simulink model "impedanceControl2012b"  (Simulink 8.0)
settings: Solver=FixedStepDiscrete  StartTime=0.0  StopTime=CONFIG.SIMULATION_TIME  FixedStep=Ts  RelTol=1e-3
InitFcn:
  | cd(fileparts(which(bdroot)));
  | init_impedanceControl;
values from neighbouring files (symbols this model uses):
  GRAV_COMP = 1    [init_impedanceControl.m]
  MOVING = 0    [init_impedanceControl.m]
undefined symbols (not defined in the file or in its folder): AMPLS, FREQS, Kd, Kp, ROBOT_DOF
libraries: WBToolboxLibrary x10
settings Model: Creator=daniele  LastModifiedBy=gnava
settings DataIOCC: SignalLoggingSaveFormat=ModelDataLogs
settings OptimizationCC: ExpressionDepthLimit=128
settings DebuggingCC: UnderspecifiedInitializationDetection=Simplified  MergeDetectMultiDrivingBlocksExec=error  MultiTaskDSMMsg=warning  MultiTaskCondExecSysMsg=none  FrameProcessingCompatibilityMsg=error  StateNameClashWarn=none  StrictBusMsg=ErrorOnBusTreatedAsVector
settings CodeAppCC: CustomSymbolStrType=$N$R$M_T
settings GRTTargetCC: CodeReplacementLibrary=C89/C90 (ANSI)

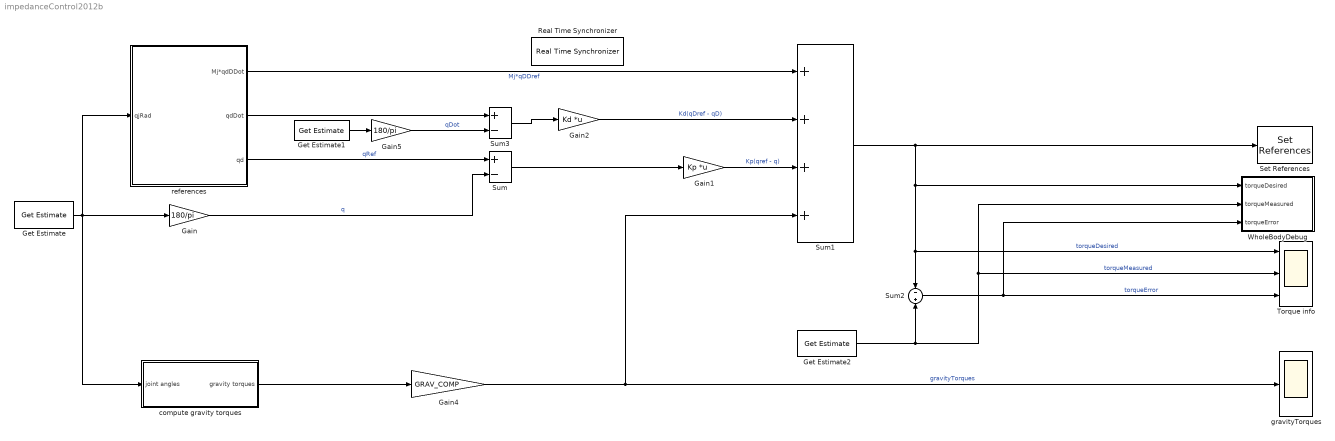
== system impedanceControl2012b ==
  Gain : Gain  Gain=180/pi
  Gain1 : Gain  Gain=Kp  Multiplication=Matrix(K*u)
  Gain2 : Gain  Gain=Kd  Multiplication=Matrix(K*u)
  Gain4 : Gain  Gain=GRAV_COMP
  Gain5 : Gain  Gain=180/pi
  Get Estimate : WBToolboxLibrary/wholeBodyStates/Get Estimate  estimateType=Joints Position  robotName=WBT_robotName  localName=WBT_modelName  wbiFile=WBT_wbiFilename  wbiList=WBT_wbiList
  Get Estimate1 : WBToolboxLibrary/wholeBodyStates/Get Estimate  estimateType=Joints Velocity  robotName=WBT_robotName  localName=WBT_modelName  wbiFile=WBT_wbiFilename  wbiList=WBT_wbiList
  Get Estimate2 : WBToolboxLibrary/wholeBodyStates/Get Estimate  estimateType=Joints Torque  robotName=WBT_robotName  localName=WBT_modelName  wbiFile=WBT_wbiFilename  wbiList=WBT_wbiList
  Real Time Synchronizer : WBToolboxLibrary/Utilities/Real Time Synchronizer  period=0.01
  Set References : WBToolboxLibrary/wholeBodyActuators/Set References  controlType=Torque  robotName=WBT_robotName  localName=WBT_modelName  wbiFile=WBT_wbiFilename  wbiList=WBT_wbiList
  Sum : Sum  Inputs=+-
  Sum1 : Sum  Inputs=++++
  Sum2 : Sum  Inputs=-|+
  Sum3 : Sum  Inputs=+-
  Torque info : Scope  NumInputPorts=3
      settings: TimeRange=20  ShowLegends=on  MaxDataPoints=5000  SaveToWorkspace=off  SaveName=ScopeData  YMin=-20.93013~-24.21652~-4.0063  YMax=5.78387~6.06845~4.66596  SampleTime=-1  DataFormat=Array
  WholeBodyDebug : Subsystem
  compute gravity torques : Subsystem
  gravityTorques : Scope
      settings: TimeRange=20  ShowLegends=on  MaxDataPoints=5000  SaveToWorkspace=off  YMin=-21.44461  YMax=11.35993  SampleTime=-1  DataFormat=Array
  references : Subsystem
  wires:
  Gain/1 -> Sum/2  "q"
  Sum/1 -> Gain1/1
  Gain1/1 -> Sum1/3  "Kp(qref - q)"
  Gain2/1 -> Sum1/2  "Kd(qDref - qD)"
  Get Estimate/1 -> compute gravity torques/1(joint angles), Gain/1, references/1(qjRad)
  Get Estimate2/1 -> WholeBodyDebug/2(torqueMeasured), Torque info/2, Sum2/2  "torqueMeasured"
  Sum2/1 -> WholeBodyDebug/3(torqueError), Torque info/3  "torqueError"
  references/3(" qd") -> Sum/1  "qRef"
  Gain5/1 -> Sum3/2  "qDot"
  Sum3/1 -> Gain2/1
  references/2(qdDot) -> Sum3/1
  references/1(Mj*qdDDot) -> Sum1/1  "Mj*qDDref"
  Gain4/1 -> Sum1/4, gravityTorques/1  "gravityTorques"
  Get Estimate1/1 -> Gain5/1
  compute gravity torques/1(gravity torques) -> Gain4/1
  Sum1/1 -> WholeBodyDebug/1(torqueDesired), Sum2/1, Torque info/1, Set References/1  "torqueDesired"

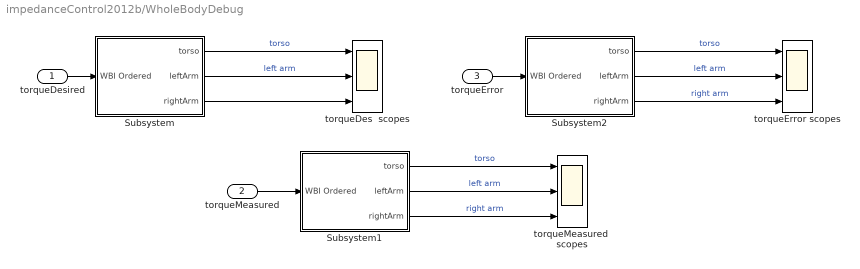
== system impedanceControl2012b/WholeBodyDebug ==
  torqueDesired : Inport
  torqueMeasured : Inport  Port=2
  torqueError : Inport  Port=3
  Subsystem : Subsystem
  Subsystem1 : Subsystem
  Subsystem2 : Subsystem
  torqueDes  scopes : Scope  NumInputPorts=3
      settings: TimeRange=60  ShowLegends=on  MaxDataPoints=5000  SaveToWorkspace=off  YMin=-21.03095~-3.42501~-3.44387  YMax=3.37527~2.67817~2.71878  SampleTime=-1
  "torqueError scopes  " : Scope  NumInputPorts=3
      settings: TimeRange=60  ShowLegends=on  MaxDataPoints=5000  SaveToWorkspace=off  SaveName=ScopeData3  YMin=-1.90536~-1.57907~-1.83653  YMax=7.25518~2.44036~2.59185  SampleTime=-1
  "torqueMeasured  scopes  " : Scope  NumInputPorts=3
      settings: TimeRange=60  ShowLegends=on  MaxDataPoints=5000  SaveToWorkspace=off  SaveName=ScopeData2  YMin=-12.98042~-3.01711~-2.9728  YMax=-3.60419~2.37899~2.11612  SampleTime=-1
  wires:
  torqueMeasured/1 -> Subsystem1/1(WBI Ordered)
  torqueError/1 -> Subsystem2/1(WBI Ordered)
  torqueDesired/1 -> Subsystem/1(WBI Ordered)
  Subsystem/1(torso) -> torqueDes  scopes/1  "torso"
  Subsystem/2(leftArm) -> torqueDes  scopes/2  "left arm"
  Subsystem1/1(torso) -> "torqueMeasured  scopes  "/1  "torso"
  Subsystem1/2(leftArm) -> "torqueMeasured  scopes  "/2  "left arm"
  Subsystem1/3(rightArm) -> "torqueMeasured  scopes  "/3  "right arm"
  Subsystem2/1(torso) -> "torqueError scopes  "/1  "torso"
  Subsystem2/2(leftArm) -> "torqueError scopes  "/2  "left arm"
  Subsystem2/3(rightArm) -> "torqueError scopes  "/3  "right arm"
  Subsystem/3(rightArm) -> torqueDes  scopes/3

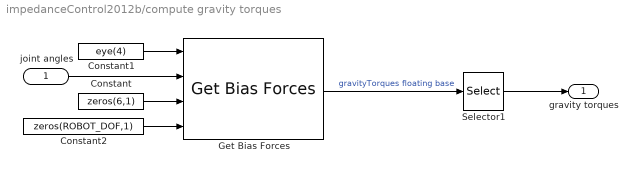
== system impedanceControl2012b/compute gravity torques ==
  joint angles : Inport
  Constant : Constant  Value=zeros(6,1)
  Constant1 : Constant  Value=eye(4)
  Constant2 : Constant  Value=zeros(ROBOT_DOF,1)
  Get Bias Forces : WBToolboxLibrary/wholeBodyModel/Dynamics/Get Bias Forces  robotName=WBT_robotName  localName=WBT_modelName  wbiFile=WBT_wbiFilename  wbiList=WBT_wbiList  explicitGravity=off
  Selector1 : Selector  InputPortWidth=ROBOT_DOF+6  IndexOptions=Index vector (dialog)  Indices=[7:ROBOT_DOF+6]  OutputSizes=1
  gravity torques : Outport
  wires:
  Selector1/1 -> gravity torques/1
  Constant1/1 -> Get Bias Forces/1
  Constant2/1 -> Get Bias Forces/4
  joint angles/1 -> Get Bias Forces/2
  Constant/1 -> Get Bias Forces/3
  Get Bias Forces/1 -> Selector1/1  "gravityTorques floating base"

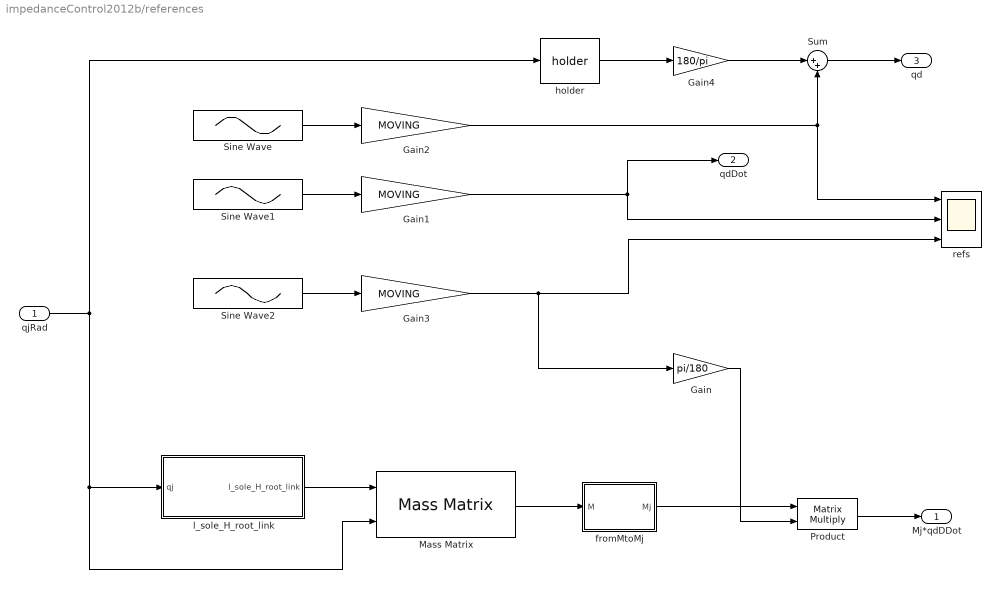
== system impedanceControl2012b/references ==
  qjRad : Inport
  Gain : Gain  Gain=pi/180
  Gain1 : Gain  Gain=MOVING
  Gain2 : Gain  Gain=MOVING
  Gain3 : Gain  Gain=MOVING
  Gain4 : Gain  Gain=180/pi
  Mass Matrix : WBToolboxLibrary/wholeBodyModel/Dynamics/Mass Matrix  robotName=WBT_robotName  localName=WBT_modelName  wbiFile=WBT_wbiFilename  wbiList=WBT_wbiList
  Product : Product  Multiplication=Matrix(*)
  Sine Wave : Sin  Amplitude=AMPLS  Frequency=FREQS*2*pi  SampleTime=0
  Sine Wave1 : Sin  Amplitude=AMPLS.*FREQS*2*pi  Frequency=FREQS*2*pi  Phase=pi/2  SampleTime=0
  Sine Wave2 : Sin  Amplitude=-AMPLS.*(FREQS*2*pi).^2  Frequency=FREQS*2*pi  SampleTime=0
  Sum : Sum  Inputs=|++
  fromMtoMj : MATLAB Function  TreatAsAtomicUnit=on
      settings: PermitHierarchicalResolution=ParametersOnly
  "holder " : WBToolboxLibrary/Utilities/holder 
  l_sole_H_root_link : Subsystem
  refs : Scope  NumInputPorts=3
      settings: TimeRange=70  ShowLegends=on  MaxDataPoints=5000  SaveToWorkspace=off  SaveName=ScopeData2  YMin=-5~-5~-5  YMax=4~5~5  SampleTime=-1  DataFormat=Array
  Mj*qdDDot : Outport
  qdDot : Outport  Port=2
  " qd" : Outport  Port=3
  wires:
  Sine Wave/1 -> Gain2/1
  Gain2/1 -> Sum/2, refs/1
  Sine Wave1/1 -> Gain1/1
  Gain1/1 -> refs/2, qdDot/1
  Sine Wave2/1 -> Gain3/1
  Product/1 -> Mj*qdDDot/1
  Mass Matrix/1 -> fromMtoMj/1(M)
  fromMtoMj/1(Mj) -> Product/1
  Gain3/1 -> refs/3, Gain/1
  Gain/1 -> Product/2
  qjRad/1 -> "holder "/1, l_sole_H_root_link/1(qj), Mass Matrix/2
  Sum/1 -> " qd"/1
  "holder "/1 -> Gain4/1
  Gain4/1 -> Sum/1
  l_sole_H_root_link/1(l_sole_H_root_link) -> Mass Matrix/1

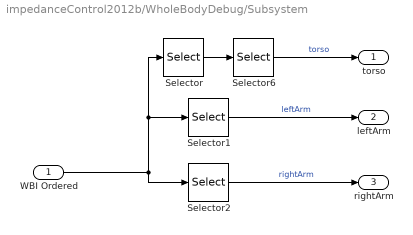
== system impedanceControl2012b/WholeBodyDebug/Subsystem ==
  WBI Ordered : Inport
  Selector : Selector  InputPortWidth=ROBOT_DOF  IndexOptions=Index vector (dialog)  Indices=[1:3]  OutputSizes=1
  Selector1 : Selector  InputPortWidth=ROBOT_DOF  IndexOptions=Index vector (dialog)  Indices=[4:7]  OutputSizes=1
  Selector2 : Selector  InputPortWidth=ROBOT_DOF  IndexOptions=Index vector (dialog)  Indices=[8:11]  OutputSizes=1
  Selector6 : Selector  InputPortWidth=3  IndexOptions=Index vector (dialog)  Indices=[3 2 1]  OutputSizes=1
  torso : Outport
  leftArm : Outport  Port=2
  rightArm : Outport  Port=3
  wires:
  Selector/1 -> Selector6/1
  Selector1/1 -> leftArm/1  "leftArm"
  Selector6/1 -> torso/1  "torso"
  Selector2/1 -> rightArm/1  "rightArm"
  WBI Ordered/1 -> Selector2/1, Selector1/1, Selector/1

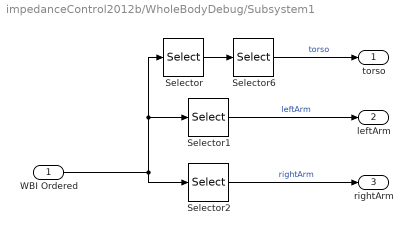
== system impedanceControl2012b/WholeBodyDebug/Subsystem1 ==
  WBI Ordered : Inport
  Selector : Selector  InputPortWidth=ROBOT_DOF  IndexOptions=Index vector (dialog)  Indices=[1:3]  OutputSizes=1
  Selector1 : Selector  InputPortWidth=ROBOT_DOF  IndexOptions=Index vector (dialog)  Indices=[4:7]  OutputSizes=1
  Selector2 : Selector  InputPortWidth=ROBOT_DOF  IndexOptions=Index vector (dialog)  Indices=[8:11]  OutputSizes=1
  Selector6 : Selector  InputPortWidth=3  IndexOptions=Index vector (dialog)  Indices=[3 2 1]  OutputSizes=1
  torso : Outport
  leftArm : Outport  Port=2
  rightArm : Outport  Port=3
  wires:
  Selector/1 -> Selector6/1
  Selector1/1 -> leftArm/1  "leftArm"
  Selector6/1 -> torso/1  "torso"
  Selector2/1 -> rightArm/1  "rightArm"
  WBI Ordered/1 -> Selector2/1, Selector1/1, Selector/1

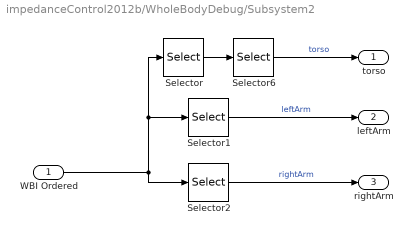
== system impedanceControl2012b/WholeBodyDebug/Subsystem2 ==
  WBI Ordered : Inport
  Selector : Selector  InputPortWidth=ROBOT_DOF  IndexOptions=Index vector (dialog)  Indices=[1:3]  OutputSizes=1
  Selector1 : Selector  InputPortWidth=ROBOT_DOF  IndexOptions=Index vector (dialog)  Indices=[4:7]  OutputSizes=1
  Selector2 : Selector  InputPortWidth=ROBOT_DOF  IndexOptions=Index vector (dialog)  Indices=[8:11]  OutputSizes=1
  Selector6 : Selector  InputPortWidth=3  IndexOptions=Index vector (dialog)  Indices=[3 2 1]  OutputSizes=1
  torso : Outport
  leftArm : Outport  Port=2
  rightArm : Outport  Port=3
  wires:
  Selector/1 -> Selector6/1
  Selector1/1 -> leftArm/1  "leftArm"
  Selector6/1 -> torso/1  "torso"
  Selector2/1 -> rightArm/1  "rightArm"
  WBI Ordered/1 -> Selector2/1, Selector1/1, Selector/1

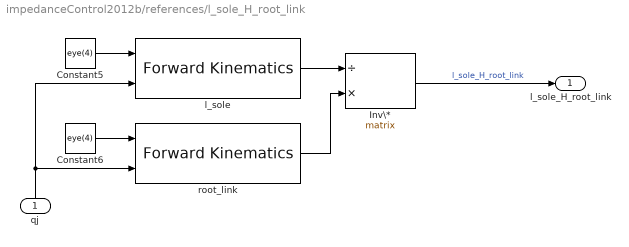
== system impedanceControl2012b/references/l_sole_H_root_link ==
  qj : Inport
  Constant5 : Constant  Value=eye(4)
  Constant6 : Constant  Value=eye(4)
  Inv\* : Product  Inputs=/*  Multiplication=Matrix(*)
  l_sole : WBToolboxLibrary/wholeBodyModel/Kinematics/Forward Kinematics  frameName='l_sole'  robotName=WBT_robotName  localName=WBT_modelName  wbiFile=WBT_wbiFilename  wbiList=WBT_wbiList
  root_link : WBToolboxLibrary/wholeBodyModel/Kinematics/Forward Kinematics  frameName='root_link'  robotName=WBT_robotName  localName=WBT_modelName  wbiFile=WBT_wbiFilename  wbiList=WBT_wbiList
  l_sole_H_root_link : Outport
  wires:
  Constant5/1 -> l_sole/1
  Inv\*/1 -> l_sole_H_root_link/1  "l_sole_H_root_link"
  l_sole/1 -> Inv\*/1
  Constant6/1 -> root_link/1
  qj/1 -> l_sole/2, root_link/2
  root_link/1 -> Inv\*/2

== matlab function references/fromMtoMj ==
  data: M input double; Mj output double
function Mj = fromMtoMj(M)
%#codegen

Mj = M(7:end,7:end);
